simulink library "calcAeroForcesInB"  (R2020a)
settings: Solver=VariableStepAuto  StartTime=0.0  StopTime=10.0  RelTol=1e-3
libraries: aerolibasang x2
settings Model: Creator=Ayaz  LastModifiedBy=Ayaz

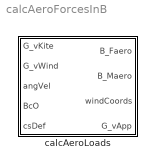
== system calcAeroForcesInB ==
  calcAeroLoads : Subsystem  mask{refChord=0.55, refSpan=5.5, refArea=3, rhoAir=1.225}
      mask prompts: refChord "Reference chord [m]"; refSpan "Reference span [m]"; refArea "Reference area [m^2]"; rhoAir "Air density"

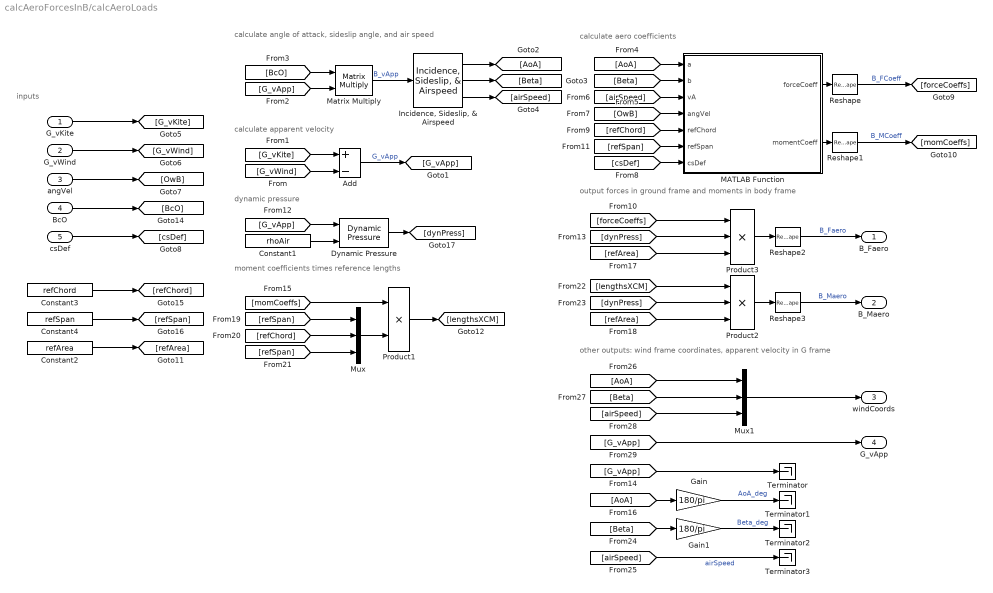
== system calcAeroForcesInB/calcAeroLoads ==
  note: other outputs: wind frame coordinates, apparent velocity in G frame
  note: output forces in ground frame and moments in body frame
  note: moment coefficients times reference lengths
  note: dynamic pressure
  note: inputs
  note: calculate angle of attack, sideslip angle, and air speed
  note: calculate aero coefficients
  note: calculate apparent velocity
  G_vKite : Inport
  G_vWind : Inport  Port=2
  angVel : Inport  Port=3
  BcO : Inport  Port=4
  csDef : Inport  Port=5
  Add : Sum  Inputs=+-
  Constant1 : Constant  Value=rhoAir
  Constant2 : Constant  Value=refArea
  Constant3 : Constant  Value=refChord
  Constant4 : Constant  Value=refSpan
  Dynamic Pressure : aerolibasang/Dynamic Pressure
  Gain : Gain  Gain=180/pi
  Gain1 : Gain  Gain=180/pi
  "Incidence, Sideslip, & Airspeed" : aerolibasang/Incidence, Sideslip, & Airspeed
  MATLAB Function : MATLAB Function  TreatAsAtomicUnit=on
  Matrix Multiply : Product  Multiplication=Matrix(*)
  Mux : Mux  Inputs=3
  Mux1 : Mux  Inputs=3
  Product1 : Product
  Product2 : Product  Inputs=3
  Product3 : Product  Inputs=3
  Reshape{,1..3} (4 alike) : Reshape  OutputDimensionality=Column vector (2-D)
  Terminator{,1..3} (4 alike) : Terminator
  B_Faero : Outport
  B_Maero : Outport  Port=2
  windCoords : Outport  Port=3
  G_vApp : Outport  Port=4
  wires:
  Product2/1 -> Reshape3/1
  [refSpan] -> MATLAB Function/6(refSpan)
  Constant4/1 -> [refSpan]
  Constant1/1 -> Dynamic Pressure/2
  [dynPress] -> Product2/2
  [refSpan] -> Mux/1
  [G_vApp] -> Dynamic Pressure/1
  [refArea] -> Product3/3
  G_vKite/1 -> [G_vKite]
  "Incidence, Sideslip, & Airspeed"/2 -> [Beta]
  Mux/1 -> Product1/2
  Constant2/1 -> [refArea]
  G_vWind/1 -> [G_vWind]
  MATLAB Function/1(forceCoeff) -> Reshape/1
  Reshape2/1 -> B_Faero/1  "B_Faero"
  Reshape1/1 -> [momCoeffs]  "B_MCoeff"
  [AoA] -> MATLAB Function/1(a)
  [lengthsXCM] -> Product2/1
  Dynamic Pressure/1 -> [dynPress]
  [refSpan] -> Mux/3
  Constant3/1 -> [refChord]
  Product1/1 -> [lengthsXCM]
  csDef/1 -> [csDef]
  Matrix Multiply/1 -> "Incidence, Sideslip, & Airspeed"/1  "B_vApp"
  Product3/1 -> Reshape2/1
  Add/1 -> [G_vApp]  "G_vApp"
  [G_vApp] -> Matrix Multiply/2
  [G_vWind] -> Add/2
  [refArea] -> Product2/3
  [momCoeffs] -> Product1/1
  [OwB] -> MATLAB Function/4(angVel)
  Reshape/1 -> [forceCoeffs]  "B_FCoeff"
  "Incidence, Sideslip, & Airspeed"/1 -> [AoA]
  [Beta] -> MATLAB Function/2(b)
  Reshape3/1 -> B_Maero/1  "B_Maero"
  [refChord] -> Mux/2
  MATLAB Function/2(momentCoeff) -> Reshape1/1
  [BcO] -> Matrix Multiply/1
  [refChord] -> MATLAB Function/5(refChord)
  "Incidence, Sideslip, & Airspeed"/3 -> [airSpeed]
  [dynPress] -> Product3/2
  [airSpeed] -> MATLAB Function/3(vA)
  [G_vKite] -> Add/1
  angVel/1 -> [OwB]
  [csDef] -> MATLAB Function/7(csDef)
  BcO/1 -> [BcO]
  [forceCoeffs] -> Product3/1
  [G_vApp] -> Terminator/1
  [AoA] -> Gain/1
  [Beta] -> Gain1/1
  Gain/1 -> Terminator1/1  "AoA_deg"
  Gain1/1 -> Terminator2/1  "Beta_deg"
  [airSpeed] -> Terminator3/1  "airSpeed"
  [AoA] -> Mux1/1
  [Beta] -> Mux1/2
  [airSpeed] -> Mux1/3
  Mux1/1 -> windCoords/1
  [G_vApp] -> G_vApp/1

== matlab function calcAeroForcesInB/calcAeroLoads/MATLAB Function ==
  data: a input; forceCoeff output; b input; vA input; angVel input; refChord input; refSpan input; csDef input; momentCoeff output
function [forceCoeff,momentCoeff] = aeroCoefficients(a,b,vA,angVel,refChord,...
    refSpan,csDef)

[forceCoeff,momentCoeff] = calcAeroCoefficients(a,b,vA,angVel,refChord,...
    refSpan,csDef);

end
